simulink model "Test_courant"  (R2020b)
settings: Solver=FixedStepAuto  StartTime=0.0  StopTime=10.0  RelTol=1e-3
undefined symbols (not defined in the file or in its folder): LL, RR
settings Model: Creator=Alexi  LastModifiedBy=Alexi

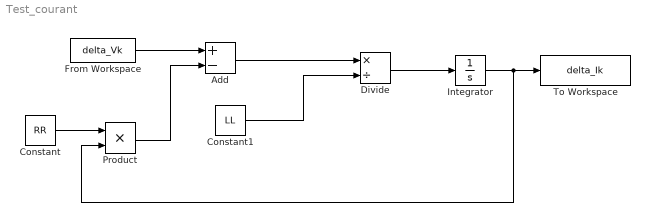
== system Test_courant ==
  Add : Sum  Inputs=+-
  Constant : Constant  Value=RR
  Constant1 : Constant  Value=LL
  Divide : Product  Inputs=*/
  From Workspace : FromWorkspace  VariableName=delta_Vk
  Integrator : Integrator
  Product : Product
  To Workspace : ToWorkspace  VariableName=delta_Ik  SaveFormat=Timeseries  SampleTime=-1
  wires:
  From Workspace/1 -> Add/1
  Constant/1 -> Product/1
  Product/1 -> Add/2
  Add/1 -> Divide/1
  Constant1/1 -> Divide/2
  Divide/1 -> Integrator/1
  Integrator/1 -> Product/2, To Workspace/1
